simulink model "Choi_Simulink"  (R2024b)
settings: Solver=VariableStepAuto  StartTime=0.0  StopTime=60  RelTol=1e-3
values from neighbouring files (symbols this model uses):
  EA_0 = deg2rad([0 0 0]')    [Choi_SimulinkScript.m]    (also in SADS_UKF_Script.m = deg2rad([10 10 0]'); pointMassTest.m = [0 0 0]')
  g_N = [0 0 -9.81]    [Choi_SimulinkScript.m]    (also in SADS_UKF_Script.m; pointMassTest.m = [0 0 -9.81]')
  J_0 = [1.815  -0.014 0.004 ... (first row only)    [Choi_SimulinkScript.m]    (also in Silva_SimulinkScript.m = [0.265 -0.014 -0.035; -0.014 0.246 -0.018; -0.035 -0.018 0.4; pointMassTest.m = diag([0.0226, 0.0257 0.0266]))
  K_I = gainScale*1    (= 0.5)    [Choi_SimulinkScript.m]
  K_omega = gainScale*3    (= 1.5)    [Choi_SimulinkScript.m]
  K_q = gainScale*1    (= 0.5)    [Choi_SimulinkScript.m]
  m_mmu = 2 * ((0.015*6) + (n*.236) + 0.177)    (= 2.894)    [Choi_SimulinkScript.m]    (also in Silva_Matlab.m = 0.7; Silva_Matlab_Implementation.m = 0.7; Silva_SimulinkScript.m = 0.7)
  m_s = 33.629    [Choi_SimulinkScript.m]    (also in SADS_UKF_Script.m; pointMassTest.m = 4.2)
  omega_0 = [0 0.0001 0]'    [Choi_SimulinkScript.m]    (also in SADS_UKF_Script.m = [0 0.00 0.00]'; Silva_SimulinkScript.m = [0 0 0.005]')
  q_0 = eul2quat(EA_0')'    [Choi_SimulinkScript.m]    (also in SADS_UKF_Script.m = eul2quat(EA_0',"XYZ")'; Silva_SimulinkScript.m = [1 0 0 0]'; pointMassTest.m = [0 0 0 1]')
  q_d = [1 0 0 0]'    [Choi_SimulinkScript.m]
  q_e_0 = [q_e_0(2) q_e_0(3) q_e_0(4)]'    [Choi_SimulinkScript.m]
  r_0 = [-6*10^-3, 7*10^-3 ,-3*10^-2]'    [Choi_SimulinkScript.m]    (also in SADS_UKF_Script.m = [-0.003 0.006 -0.001]')
libraries: sharedtransform x1
settings Model: Creator=camer  LastModifiedBy=camer

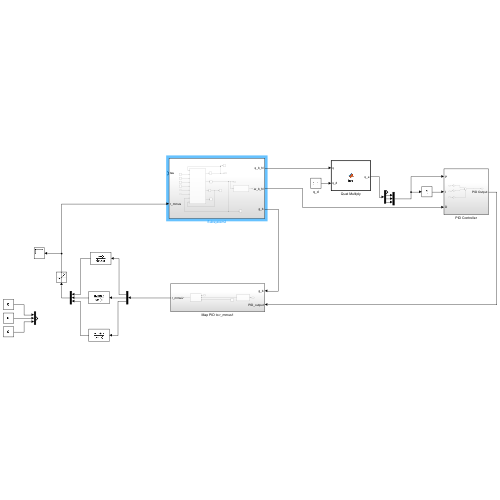
[thumbnail: Simulink's stored preview of the top-level diagram]
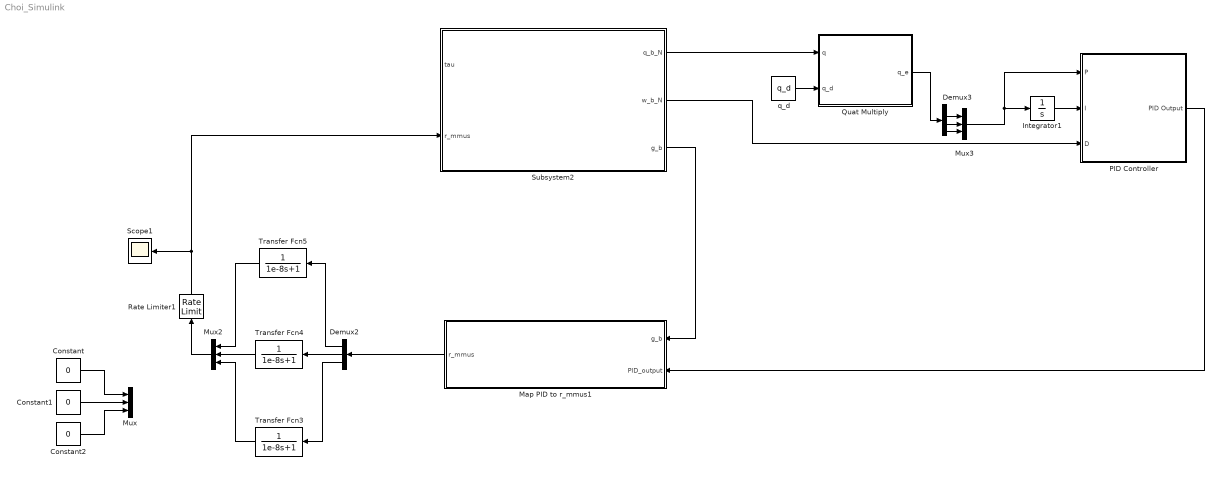
== system Choi_Simulink ==
  Constant : Constant  Value=0
  Constant1 : Constant  Value=0
  Constant2 : Constant  Value=0
  Demux2 : Demux  Outputs=3
  Demux3 : Demux
  Integrator1 : Integrator  InitialCondition=q_e_0
  Map PID to r_mmus1 : Subsystem
  Mux : Mux  Inputs=3
  Mux2 : Mux  Inputs=3
  Mux3 : Mux  Inputs=3
  PID Controller : Subsystem
  Quat Multiply : MATLAB Function  TreatAsAtomicUnit=on
  Rate Limiter1 : RateLimiter  RisingSlewLimit=0.030  FallingSlewLimit=-0.030  SampleTimeMode=inherited
  Scope1 : Scope
  Subsystem2 : Subsystem
  Transfer Fcn3 : TransferFcn  Denominator=[1e-8 1]
  Transfer Fcn4 : TransferFcn  Denominator=[1e-8 1]
  Transfer Fcn5 : TransferFcn  Denominator=[1e-8 1]
  q_d : Constant  Value=q_d
  wires:
  Quat Multiply/1(q_e) -> Demux3/1
  Mux2/1 -> Rate Limiter1/1
  Subsystem2/1(q_b_N) -> Quat Multiply/1(q)
  Subsystem2/3(g_b) -> Map PID to r_mmus1/1(g_b)
  Integrator1/1 -> PID Controller/2(I)
  q_d/1 -> Quat Multiply/2(q_d)
  Rate Limiter1/1 -> Subsystem2/2(r_mmus), Scope1/1
  Subsystem2/2(w_b_N) -> PID Controller/3(D)
  Mux3/1 -> PID Controller/1(P), Integrator1/1
  Demux2/3 -> Transfer Fcn3/1
  Demux3/2 -> Mux3/1
  Demux3/4 -> Mux3/3
  PID Controller/1(PID Output) -> Map PID to r_mmus1/2(PID_output)
  Demux2/2 -> Transfer Fcn4/1
  Map PID to r_mmus1/1(r_mmus) -> Demux2/1
  Demux2/1 -> Transfer Fcn5/1
  Demux3/3 -> Mux3/2
  Transfer Fcn5/1 -> Mux2/1
  Transfer Fcn4/1 -> Mux2/2
  Transfer Fcn3/1 -> Mux2/3
  Constant/1 -> Mux/1
  Constant1/1 -> Mux/2
  Constant2/1 -> Mux/3

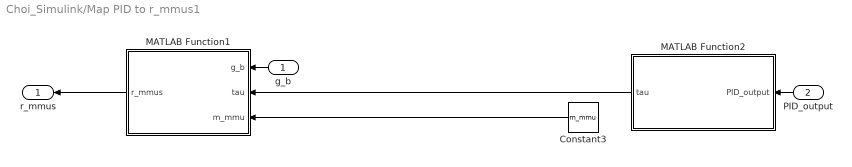
== system Choi_Simulink/Map PID to r_mmus1 ==
  g_b : Inport
  PID_output : Inport  Port=2
  Constant3 : Constant  Value=m_mmu
  MATLAB Function1 : MATLAB Function  TreatAsAtomicUnit=on
  MATLAB Function2 : MATLAB Function  TreatAsAtomicUnit=on
  r_mmus : Outport
  wires:
  PID_output/1 -> MATLAB Function2/1(PID_output)
  MATLAB Function2/1(tau) -> MATLAB Function1/2(tau)
  Constant3/1 -> MATLAB Function1/3(m_mmu)
  g_b/1 -> MATLAB Function1/1(g_b)
  MATLAB Function1/1(r_mmus) -> r_mmus/1

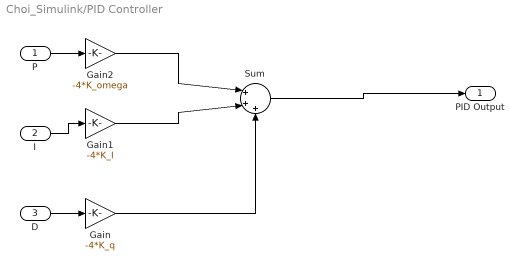
== system Choi_Simulink/PID Controller ==
  P : Inport
  I : Inport  Port=2
  D : Inport  Port=3
  Gain : Gain  Gain=-4*K_q
  Gain1 : Gain  Gain=-4*K_I
  Gain2 : Gain  Gain=-4*K_omega
  Sum : Sum  Inputs=|+++
  PID Output : Outport
  wires:
  Gain2/1 -> Sum/1
  P/1 -> Gain2/1
  Gain/1 -> Sum/3
  D/1 -> Gain/1
  Gain1/1 -> Sum/2
  Sum/1 -> PID Output/1
  I/1 -> Gain1/1

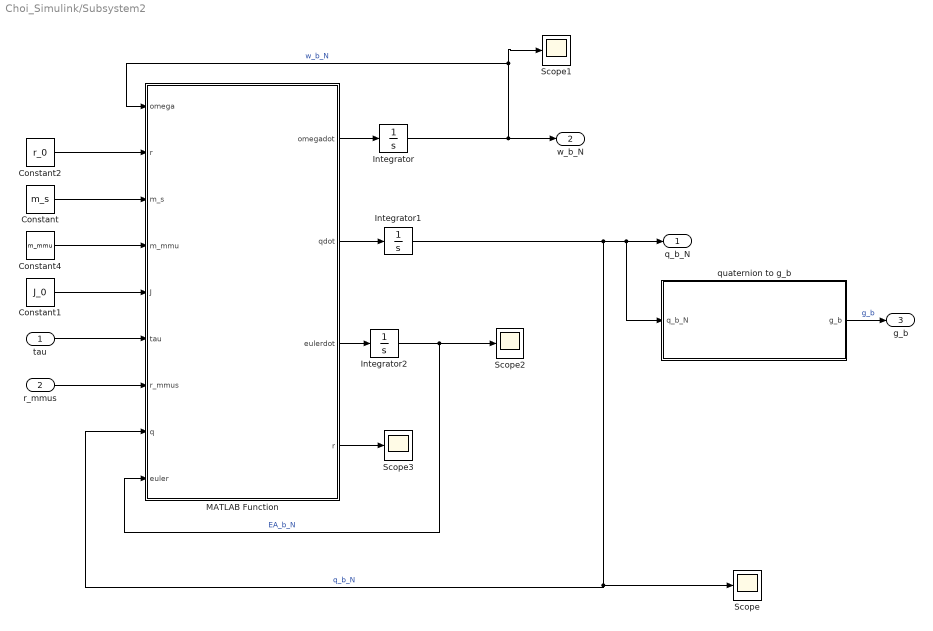
== system Choi_Simulink/Subsystem2 ==
  tau : Inport
  r_mmus : Inport  Port=2
  Constant : Constant  Value=m_s
  Constant1 : Constant  Value=J_0
  Constant2 : Constant  Value=r_0
  Constant4 : Constant  Value=m_mmu
  Integrator : Integrator  InitialCondition=omega_0
  Integrator1 : Integrator  InitialCondition=q_0
  Integrator2 : Integrator  InitialCondition=EA_0
  MATLAB Function : MATLAB Function  TreatAsAtomicUnit=on
  Scope{,1..3} (4 alike) : Scope
  quaternion to g_b : Subsystem
  q_b_N : Outport
  w_b_N : Outport  Port=2
  g_b : Outport  Port=3
  wires:
  MATLAB Function/4(r) -> Scope3/1
  Integrator/1 -> Scope1/1, MATLAB Function/1(omega), w_b_N/1  "w_b_N"
  Constant4/1 -> MATLAB Function/4(m_mmu)
  Constant1/1 -> MATLAB Function/5(J)
  Constant2/1 -> MATLAB Function/2("r ")
  Constant/1 -> MATLAB Function/3(m_s)
  tau/1 -> MATLAB Function/6(tau)
  Integrator1/1 -> quaternion to g_b/1(q_b_N), q_b_N/1, MATLAB Function/8(q), Scope/1  "q_b_N"
  MATLAB Function/2(qdot) -> Integrator1/1
  MATLAB Function/1(omegadot) -> Integrator/1
  r_mmus/1 -> MATLAB Function/7(r_mmus)
  quaternion to g_b/1(g_b) -> g_b/1  "g_b"
  MATLAB Function/3(eulerdot) -> Integrator2/1
  Integrator2/1 -> Scope2/1, MATLAB Function/9(euler)  "EA_b_N"

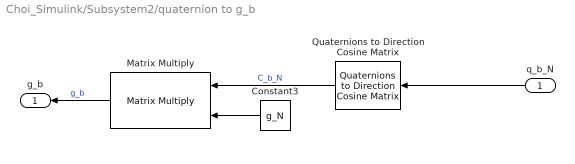
== system Choi_Simulink/Subsystem2/quaternion to g_b ==
  q_b_N : Inport
  Constant3 : Constant  Value=g_N
  Matrix Multiply : Product  Multiplication=Matrix(*)
  Quaternions to Direction Cosine Matrix : sharedtransform/Quaternions to  Direction Cosine Matrix  aMode=aMode
  g_b : Outport
  wires:
  Constant3/1 -> Matrix Multiply/2
  Quaternions to Direction Cosine Matrix/1 -> Matrix Multiply/1  "C_b_N"
  q_b_N/1 -> Quaternions to Direction Cosine Matrix/1
  Matrix Multiply/1 -> g_b/1  "g_b"

== matlab function Choi_Simulink/Map PID to r_mmus1/MATLAB Function1 ==
  data: g_b input; tau input; r_mmus output; m_mmu input
function r_mmus = fcn(g_b,tau,m_mmu)

    g_b_cross = [0 -g_b(3) g_b(2);
               g_b(3) 0 -g_b(1);
              -g_b(2) g_b(1) 0];

r_mmus = (g_b_cross*tau)./(norm(g_b)^2*m_mmu);

== matlab function Choi_Simulink/Map PID to r_mmus1/MATLAB Function2 ==
  data: PID_output input; tau output
function tau = fcn(PID_output)

tau = [PID_output(1) PID_output(2) 0]';

== matlab function Choi_Simulink/Quat Multiply ==
  data: q input; q_e output; q_d input
function q_e = fcn(q,q_d)

q_e = [q_d(1) -q_d(2) -q_d(3) -q_d(4);
       q_d(2)  q_d(1) -q_d(4)  q_d(3);
       q_d(3)  q_d(4)  q_d(1) -q_d(2);
       q_d(4) -q_d(3)  q_d(2)  q_d(1);]*q;

== matlab function Choi_Simulink/Subsystem2/MATLAB Function ==
  data: omega input; r input; m_s input; m_mmu input; J input; tau input; r_mmus input; omegadot output; q input; qdot output; eulerdot output; r output; euler input
function [omegadot, qdot,eulerdot,r] = fcn(omega,r,m_s,m_mmu,J,tau,r_mmus,q,euler)
% Equations of motion developed in the work of Chesi.

g = 9.81; % 

% Gravity vector in body-frame
C_N_b = [2*q(1)^2-1+2*q(2)^2 2*q(2)*q(3)-2*q(1)*q(4) 2*q(2)*q(4)+2*q(1)*q(3);
       2*q(2)*q(3)+2*q(1)*q(4) 2*q(1)^2-1+2*q(3)^2 2*q(3)*q(4)-2*q(1)*q(2);
       2*q(2)*q(4)-2*q(1)*q(3) 2*q(3)*q(4)+2*q(1)*q(2) 2*q(1)^2-1+2*q(4)^2];

g_b = C_N_b' * [0; 0; -g];

u = [1 0 0; % column vectors that each mass slides along
     0 1 0;
     0 0 1];

sum = zeros(size(u,2), 1);
for i = 1:size(u,2)
    sum = sum + m_mmu*r_mmus(i)*u(:,i);
end

r_new = r + (1/m_s).*sum;
r = r_new;

% Equations of Motion
omegadot=J\(-cross(omega,J*omega)+cross(r,g_b*m_s));

% Quaternion rates
qdot = 0.5*[0 -omega(1) -omega(2) -omega(3);
             omega(1) 0 omega(3) -omega(2);
             omega(2) -omega(3) 0 omega(1);
             omega(3) omega(2) -omega(1) 0]*q;

% Euler rates
Phi = euler(1);
Theta = euler(2);
Psi = euler(3);

matrix = (1/cos(Theta)).*[cos(Theta) sin(Phi)*sin(Theta)  cos(Phi)*sin(Theta);
                              0          cos(Phi)*cos(Theta) -sin(Phi)*cos(Theta);
                              0          sin(Phi)             cos(Phi)];

product = matrix * omega;

dPhi = product(1);
dTheta = product(2);
dPsi = product(3);

eulerdot = [dPhi dTheta dPsi]';
